simulink model "model1"  (R2025b)
settings: Solver=FixedStepAuto  StartTime=0.0  StopTime=10.0  RelTol=1e-3
settings Model: DataDictionary=model1.sldd  Creator=eren  LastModifiedBy=eren
settings OptimizationCC: DefaultParameterBehavior=Inlined  UseDivisionForNetSlopeComputation=on  GainParamInheritBuiltInType=on  UseFloatMulNetSlope=on  InlineInvariantSignals=on  PassReuseOutputArgsAs=Individual arguments  ZeroExternalMemoryAtStartup=off  ZeroInternalMemoryAtStartup=off  NoFixptDivByZeroProtection=on  EfficientFloat2IntCast=on  LifeSpan=1  OptimizeBlockOrder=speed  DifferentSizesBufferReuse=on  EfficientTunableParamExpr=on
settings DebuggingCC: ParameterTunabilityLossMsg=error
settings HardwareCC: ProdBitPerPointer=32.0  ProdBitPerSizeT=32.0  ProdBitPerPtrDiffT=32.0  ProdLargestAtomicInteger=Long  ProdLargestAtomicFloat=Double  ProdWordSize=32.0  ProdLongLongMode=on  ProdHWDeviceType=ARM Compatible->ARM Cortex-M
settings SFSimCC: MATLABDynamicMemAlloc=off
settings RTWCC: SystemTargetFile=ert.tlc  TemplateMakefile=ert_default_tmf  Description=Embedded Coder
settings CodeAppCC: ForceParamTrailComments=on  IgnoreCustomStorageClasses=off  OperatorAnnotations=on  SimulinkDataObjDesc=on  SFDataObjDesc=on  CustomSymbolStrGlobalVar=rt$N$M  CustomSymbolStrType=$N$M  CustomSymbolStrFcn=$N$M$F  CustomSymbolStrMacro=$N$M  InsertBlockDesc=on
settings ERTTargetCC: ERTCustomFileTemplate=example_file_process.tlc  ERTFilePackagingFormat=CompactWithDataFile  TargetLangStandard=C99 (ISO)  GenerateSampleERTMain=on  IncludeMdlTerminateFcn=off  CombineSignalStateStructs=on  SupportAbsoluteTime=off  PurelyIntegerCode=on  SupportNonFinite=off  SupportComplex=off  SupportContinuousTime=on

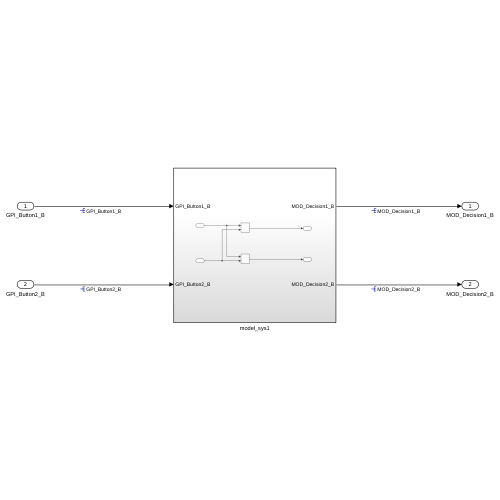
[thumbnail: Simulink's stored preview of the top-level diagram]
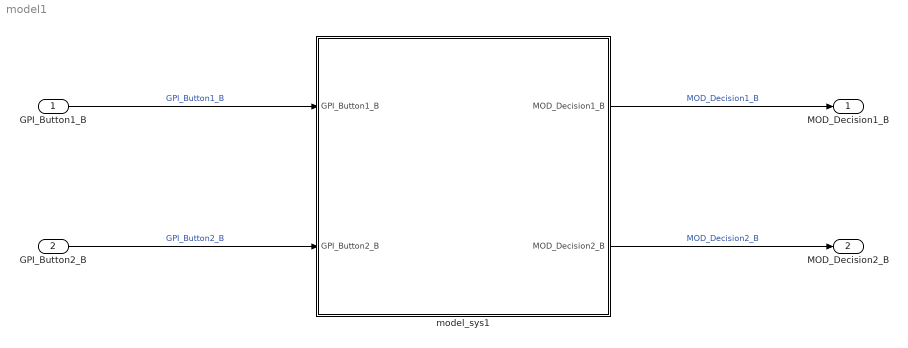
== system model1 ==
  GPI_Button1_B : Inport
  GPI_Button2_B : Inport  Port=2
  model_sys1 : Subsystem
  MOD_Decision1_B : Outport
  MOD_Decision2_B : Outport  Port=2
  wires:
  GPI_Button1_B/1 -> model_sys1/1(GPI_Button1_B)  "GPI_Button1_B"
  GPI_Button2_B/1 -> model_sys1/2(GPI_Button2_B)  "GPI_Button2_B"
  model_sys1/1(MOD_Decision1_B) -> MOD_Decision1_B/1  "MOD_Decision1_B"
  model_sys1/2(MOD_Decision2_B) -> MOD_Decision2_B/1  "MOD_Decision2_B"

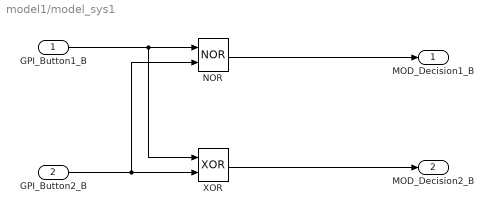
== system model1/model_sys1 ==
  GPI_Button1_B : Inport
  GPI_Button2_B : Inport  Port=2
  NOR : Logic  Operator=NOR  AllPortsSameDT=off  OutDataTypeStr=boolean
  XOR : Logic  Operator=XOR  AllPortsSameDT=off  OutDataTypeStr=boolean
  MOD_Decision1_B : Outport
  MOD_Decision2_B : Outport  Port=2
  wires:
  GPI_Button1_B/1 -> XOR/1, NOR/1
  GPI_Button2_B/1 -> XOR/2, NOR/2
  NOR/1 -> MOD_Decision1_B/1
  XOR/1 -> MOD_Decision2_B/1
